simulink model "del2_sensors"  (R2024a)
settings: Solver=VariableStepAuto  StartTime=0.0  StopTime=inf  MaxStep=1e-3  MinStep=1e-5  RelTol=1e-4
InitFcn:
  | id_setup()
StartFcn:
  | c_id = evalin('base', "car_id");
  | g_id = evalin('base', "group_id");
  | mqttBasic(c_id,g_id);
libraries: read x2, instrumentlib x1, init x1
settings Model: Creator=adriaeik  LastModifiedBy=adriaeik
settings DebuggingCC: UnderSpecifiedDimensionMsg=warning

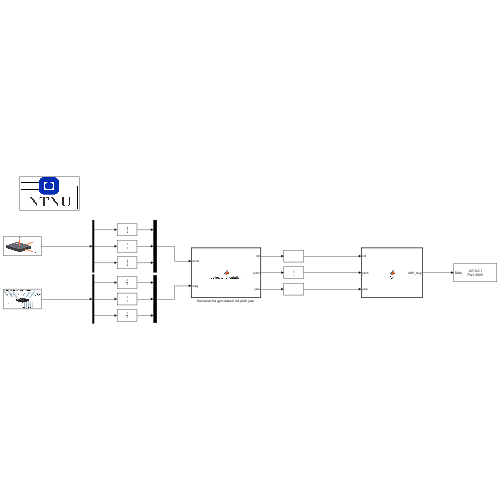
[thumbnail: Simulink's stored preview of the top-level diagram]
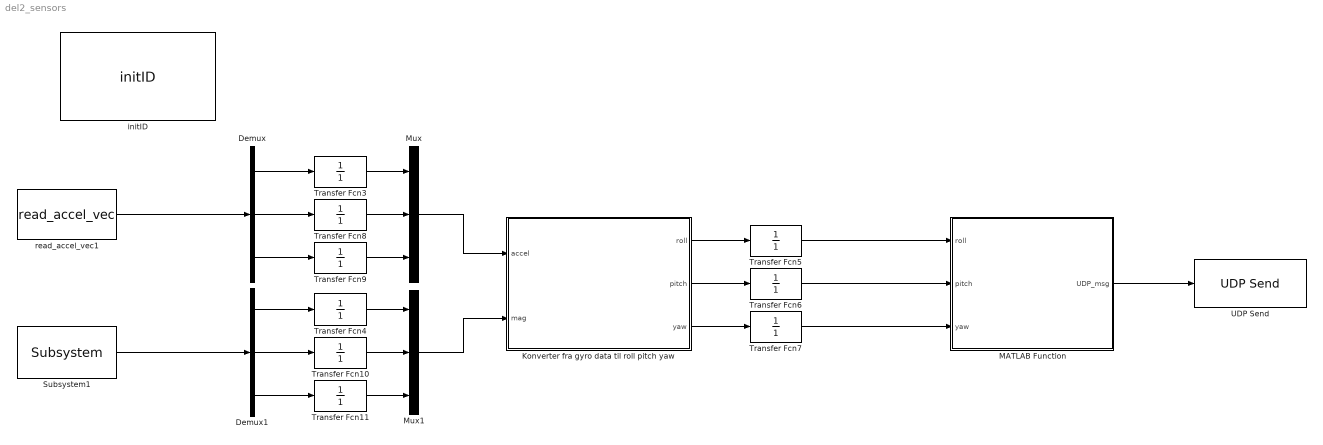
== system del2_sensors ==
  Demux : Demux  Outputs=3
  Demux1 : Demux  Outputs=3
  "Konverter fra gyro data til roll pitch yaw " : MATLAB Function  TreatAsAtomicUnit=on
  MATLAB Function : MATLAB Function  TreatAsAtomicUnit=on
  Mux : Mux  Inputs=3
  Mux1 : Mux  Inputs=3
  Subsystem1 : read/Subsystem
  Transfer Fcn{3..11} (9 alike) : TransferFcn  Denominator=[0 1]
  UDP Send : instrumentlib/UDP Send  Host=127.0.0.1  Port=5005  LocalAddress=0.0.0.0  LocalPort=-1  EnablePortSharing=off  OutputDatagramPacketSize=8  ByteOrder=big-endian  EnableBlockingMode=on  SimulateUsing=Interpreted execution
  initID : init/initID  carID=99  groupID=99
  read_accel_vec1 : read/read_accel_vec
  wires:
  Mux/1 -> "Konverter fra gyro data til roll pitch yaw "/1(accel)
  read_accel_vec1/1 -> Demux/1
  Subsystem1/1 -> Demux1/1
  "Konverter fra gyro data til roll pitch yaw "/1(roll) -> Transfer Fcn5/1
  "Konverter fra gyro data til roll pitch yaw "/3(yaw) -> Transfer Fcn7/1
  "Konverter fra gyro data til roll pitch yaw "/2(pitch) -> Transfer Fcn6/1
  Transfer Fcn5/1 -> MATLAB Function/1(roll)
  Transfer Fcn6/1 -> MATLAB Function/2(pitch)
  Transfer Fcn7/1 -> MATLAB Function/3(yaw)
  MATLAB Function/1(UDP_msg) -> UDP Send/1
  Transfer Fcn9/1 -> Mux/3
  Demux/3 -> Transfer Fcn9/1
  Demux/2 -> Transfer Fcn8/1
  Demux/1 -> Transfer Fcn3/1
  Transfer Fcn3/1 -> Mux/1
  Transfer Fcn8/1 -> Mux/2
  Demux1/3 -> Transfer Fcn11/1
  Transfer Fcn11/1 -> Mux1/3
  Demux1/2 -> Transfer Fcn10/1
  Transfer Fcn10/1 -> Mux1/2
  Transfer Fcn4/1 -> Mux1/1
  Demux1/1 -> Transfer Fcn4/1
  Mux1/1 -> "Konverter fra gyro data til roll pitch yaw "/2(mag)

== matlab function del2_sensors/MATLAB Function ==
  data: roll input; pitch input; yaw input; UDP_msg output size=[8 1]
function UDP_msg = fcn(roll, pitch, yaw)

R_bw = eul2rotm([yaw, pitch, roll], 'ZYX'); 

z_vec = [0; 0; 1]; 

Rot_joystick = R_bw * z_vec; 



y = Rot_joystick(1);
x = Rot_joystick(2); 


%Ikke tenk på det
xy_single = single([x; y]);
xy_be     = swapbytes(xy_single);

UDP_msg = typecast(xy_be, 'uint8');

== matlab function del2_sensors/Konverter fra gyro data til roll pitch yaw  ==
  data: accel input; roll output; mag input; pitch output; yaw output
function [roll, pitch, yaw] = estimate_orientation(accel, mag)
%#codegen

% accel, gyro, mag: [3x1] sensorvektorar
% gyro(3) er yaw i radianar (allerede integrert)

% --- Normaliser og formater ---
accel = accel(:); accel = accel / norm(accel);
mag   = mag(:);   mag = mag / norm(mag);


% --- Estimer roll og pitch frå akselerometer ---

% _____________________________________________________________
%%%%%%%%%%%%%%%%%%%%%%%% HER SKAL DERE ENDRE %%%%%%%%%%%%%%%%%%

ax = accel(1);
ay = accel(2);
az = accel(3);





% Regn ut selv! 

raw_pitch = 0;
raw_roll  = 0;





%Hint: raw_pitch og raw roll er ikke lik 0. 
%Hint: bruk ax, ay, az. Disse er akselerasjonene i de forskjellige 
%      retningene. Finn ut hva de betyr ved å se på dataen!
%Hint: kan være lurt å tegne opp! 
%Hint: Lurt å samarbeide
%Hint: Løsningsforslaget kommer etterhvert, men hvis dere klarer å løse
%      det får dere bonuspoeng :) 
%Hint: Les oppgaveteksten

% _____________________________________________________________




% --- Tiltkompensasjon av magnetometer ---
Rx = [1 0 0;
      0 cos(raw_roll) -sin(raw_roll);
      0 sin(raw_roll)  cos(raw_roll)];
Ry = [cos(raw_pitch) 0 sin(raw_pitch);
      0 1 0;
     -sin(raw_pitch) 0 cos(raw_pitch)];

R = Ry * Rx;
mag_flat = R' * mag;  % kompenser for tilt
raw_yaw = atan2(-mag_flat(2), mag_flat(1));


roll = raw_roll; 
pitch = raw_pitch; 
yaw = raw_yaw;
